simulink model "Param_Est_P1"  (R2019b)
settings: Solver=VariableStepAuto  StartTime=0.0  StopTime=50  RelTol=1e-3
undefined symbols (not defined in the file): sigbuilder_block
libraries: simulink x1
settings Model: Creator=Kevin  LastModifiedBy=Kevin

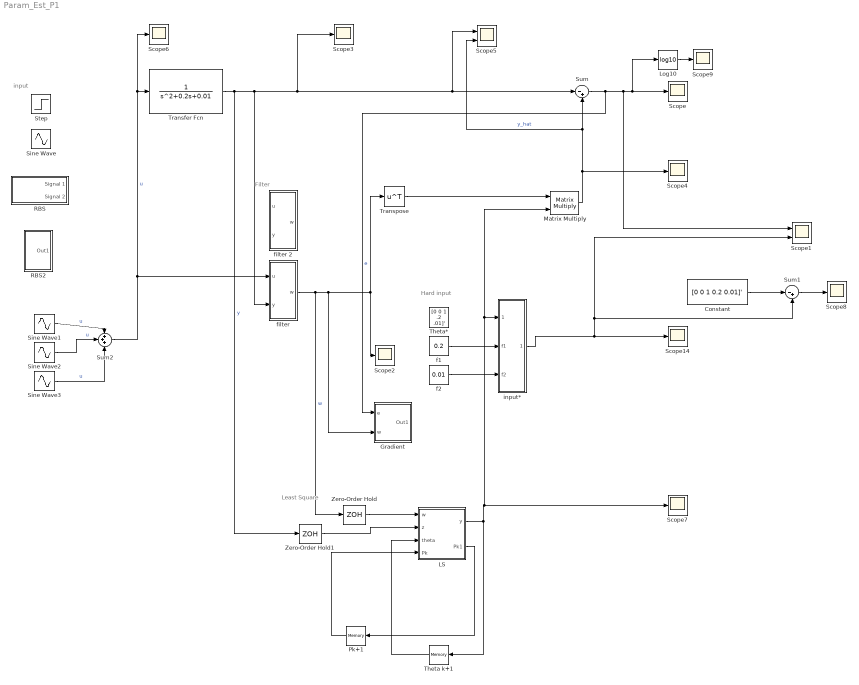
== system Param_Est_P1 ==
  note: Filter
  note: Least Square
  note: Hard input
  note: input
  Constant : Constant  Value=[0 0 1 0.2 0.01]'
  Gradient : Subsystem
  LS : MATLAB Function  TreatAsAtomicUnit=on
  Log10 : Math  Operator=log10  SignedPower=off  SaturateOnIntegerOverflow=on
  Matrix Multiply : Product  Multiplication=Matrix(*)
  Pk+1 : Memory  InitialCondition=(10^5)*eye(5)
  "RBS " : Subsystem  Tag=STV Subsys  LoadFcn=sigbuilder_block('load');  StartFcn=sigbuilder_block('start');  StopFcn=sigbuilder_block('stop');  ClipboardFcn=sigbuilder_block('clipboard');  mask(Sigbuilder block){tuvar=[0:10]}
      mask help: Simulink:masks:SigbuilderBlock_MD
      mask init:
      | if ~strcmp(get_param(bdroot(gcbh),'SimulationStatus'),'stopped') tuvar = sigbuilder_block('maskInit'); end
      settings: CopyFcn=sigbuilder_block('copy');  DeleteFcn=sigbuilder_block('delete');  ModelCloseFcn=sigbuilder_block('modelClose');  PreSaveFcn=sigbuilder_block('preSave');  PauseFcn=sigbuilder_block('pause');  ContinueFcn=sigbuilder_block('continue');  NameChangeFcn=sigbuilder_block('namechange');  OpenFcn=sigbuilder_block('open',[215 62.5 550.5 362.5 ]);  CloseFcn=sigbuilder_block('close');
      mask Display: plot(0, 0, 100, 100,[2, 2, 32, 32, 2], [68, 8, 8, 68, 68],[32, 2], [38, 38], [32, 19, 2],[53, 60, 44], [32, 17, 17, 2],[16, 16, 31, 31]);txt = getActiveGroup(gcbh);text(2, 100, txt,'verticalAlignment', 'top');
  RBS2 : Subsystem
  Scope{,2..4,6..9,14} (9 alike) : Scope
  Scope1 : Scope  NumInputPorts=2
  Scope5 : Scope  NumInputPorts=2
  Sine Wave : Sin  Frequency=0.1  SampleTime=0
  Sine Wave1 : Sin  Frequency=0.1  Phase=0.1  SampleTime=0
  Sine Wave2 : Sin  SampleTime=0
  Sine Wave3 : Sin  Frequency=2  SampleTime=0
  Step : Step  SampleTime=0
  Sum : Sum  Inputs=|-+
  Sum1 : Sum  Inputs=|-+
  Sum2 : Sum  Inputs=+++
  Theta k+1 : Memory  InitialCondition=[0 0 0 0 0]'
  Theta* : Constant  Value=[0 0 1 .2 .01]'
  Transfer Fcn : TransferFcn  Denominator=[1 ,0.2 ,0.01]
  Transpose : Math  Operator=transpose  SignedPower=off  SaturateOnIntegerOverflow=on
  Zero-Order Hold : ZeroOrderHold  SampleTime=-1
  Zero-Order Hold1 : ZeroOrderHold  SampleTime=-1
  f1 : Constant  Value=0.2
  f2 : Constant  Value=0.01
  "filter " : Subsystem
  filter 2 : Subsystem
  input* : Subsystem
  wires:
  "filter "/1(w) -> Zero-Order Hold/1, Gradient/2(w), Scope2/1, Transpose/1  "w"
  Matrix Multiply/1 -> Sum/2, Scope5/2, Scope4/1  "y_hat"
  Sum/1 -> Gradient/1(e), Scope1/1, Log10/1, Scope/1  "e"
  Transpose/1 -> Matrix Multiply/1
  f1/1 -> input*/2(f1)
  f2/1 -> input*/3(f2)
  Zero-Order Hold/1 -> LS/1(w)
  LS/1(y) -> Theta k+1/1, Matrix Multiply/2, input*/1(theta), Scope7/1
  Theta k+1/1 -> LS/3(theta)
  Pk+1/1 -> LS/4(Pk)
  LS/2(Pk1) -> Pk+1/1
  Transfer Fcn/1 -> Zero-Order Hold1/1, "filter "/2("y "), Scope5/1, Sum/1, Scope3/1  "y"
  Zero-Order Hold1/1 -> LS/2(z)
  Sum2/1 -> Transfer Fcn/1, Scope6/1, "filter "/1("u ")  "u"
  input*/1(Out1) -> Sum1/2, Scope1/2, Scope14/1
  Constant/1 -> Sum1/1
  Sum1/1 -> Scope8/1
  Sine Wave1/1 -> Sum2/1  "u"
  Sine Wave2/1 -> Sum2/2  "u"
  Sine Wave3/1 -> Sum2/3  "u"
  Log10/1 -> Scope9/1

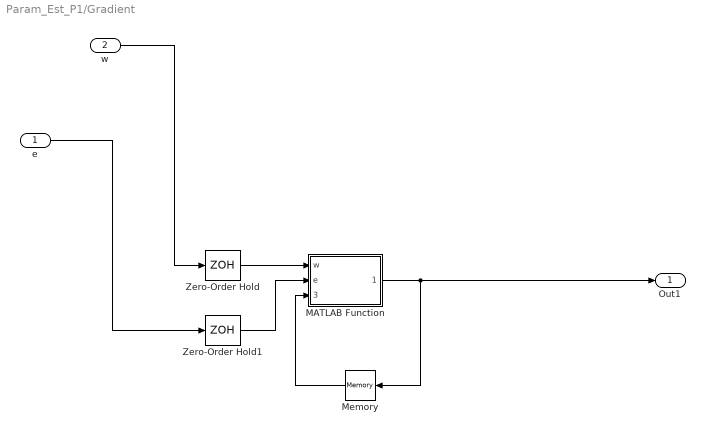
== system Param_Est_P1/Gradient ==
  e : Inport
  w : Inport  Port=2
  MATLAB Function : MATLAB Function  TreatAsAtomicUnit=on
  Memory : Memory  InitialCondition=[0 0 0.9 0.000001 0.0000001]'
  Zero-Order Hold : ZeroOrderHold  SampleTime=0.01
  Zero-Order Hold1 : ZeroOrderHold  SampleTime=0.01
  Out1 : Outport
  wires:
  MATLAB Function/1(theta_k1) -> Memory/1, Out1/1
  Zero-Order Hold/1 -> MATLAB Function/1(w)
  w/1 -> Zero-Order Hold/1
  Zero-Order Hold1/1 -> MATLAB Function/2(e)
  e/1 -> Zero-Order Hold1/1
  Memory/1 -> MATLAB Function/3(theta_1)

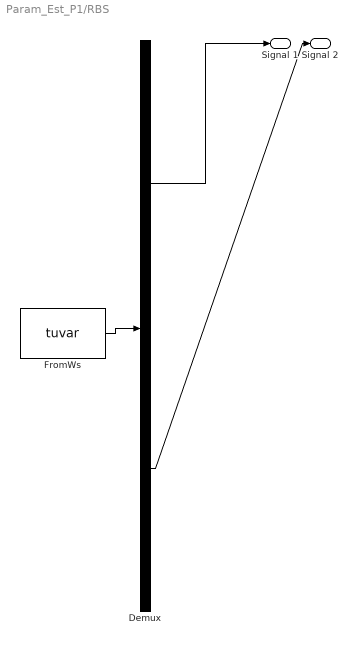
== system Param_Est_P1/RBS  ==
  Demux : Demux  Tag=STV Demux  Outputs=2
  FromWs : FromWorkspace  Tag=STV FromWs  VariableName=tuvar  SampleTime=0
      SigBuilderData=|
      | common.afterFinalStr = 'Extrapolate'
      | common.sampleTime = 0
      | dataSet.timeRange = [0 10]
      | dataSet.name = 'Group 1'
      | sbobj.Groups.Name = 'Group 1'
      | sbobj.Groups.Signals(1).Name = 'Signal 1'
      | sbobj.Groups.Signals(1).XData = [0 4 4 6 6 10]
      | sbobj.Groups.Signals(1).YData = [0 0 1 1 0 0]
      | sbobj.Groups.Signals(2).Name = 'Signal 2'
      | sbobj.Groups.Signals(2).XData = [0 0.2 0.2 0.3 0.3 0.5 0.5 0.7 0.7 1 1 1.1 1.1 1.3 1.3 1.4 1.4 1.5 1.5 1.7 1.7 2.1 2.1 2.2 2.2 2.7 2.7 2.8 2.8 2.9 2.9 3 3 3.1 3.1 3.5 3.5 3.7 3.7 3.8 3.8 3.9 3.9 4.2 4.2 4.4 4.4 4.7 4.7 5 5 5.1 5.1 5.3 5.3 5.6 5.6 5.7 5.7 5.8 5.8 5.9 5.9 6 6 6.1 6.1 6.2 6.2 6.7 6.7 7 7 7.1 7.1 7.2 7.2 7.3 7.3 7.4 7.4 7.5 7.5 7.8 7.8 7.9 7.9 8.1 8.1 8.5 8.5 8.6 8.6 8.8 8.8 8.9 8.9 9 9 9.2 9.2 9.5 9.5 9.6 9.6 9.7 9.7 10]
      | sbobj.Groups.Signals(2).YData = [1 1 0 0 1 1 0 0 1 1 0 0 1 1 0 0 1 1 0 0 1 1 0 0 1 1 0 0 1 1 0 0 1 1 0 0 1 1 0 0 1 1 0 0 1 1 0 0 1 1 0 0 1 1 0 0 1 1 0 0 1 1 0 0 1 1 0 0 1 1 0 0 1 1 0 0 1 1 0 0 1 1 0 0 1 1 0 0 1 1 0 0 1 1 0 0 1 1 0 0 1 1 0 0 1 1 0 0]
  Signal 1 : Outport  Tag=STV Outport
  Signal 2 : Outport  Tag=STV Outport  Port=2
  wires:
  Demux/1 -> Signal 1/1
  FromWs/1 -> Demux/1
  Demux/2 -> Signal 2/1

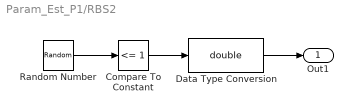
== system Param_Est_P1/RBS2 ==
  Compare To Constant : simulink/Logic and Bit Operations/Compare To Constant  relop=<=  const=1  OutDataTypeStr=boolean
  Data Type Conversion : DataTypeConversion  OutDataTypeStr=double
  Random Number : RandomNumber  Mean=1  SampleTime=10
  Out1 : Outport
  wires:
  Random Number/1 -> Compare To Constant/1
  Compare To Constant/1 -> Data Type Conversion/1
  Data Type Conversion/1 -> Out1/1

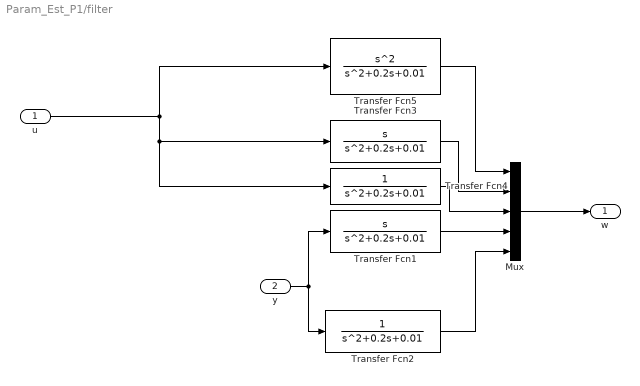
== system Param_Est_P1/filter  ==
  "u " : Inport
  "y " : Inport  Port=2
  Mux : Mux  Inputs=5
  Transfer Fcn1 : TransferFcn  Numerator=[1 0]  Denominator=[1 0.2 0.01]
  Transfer Fcn2 : TransferFcn  Denominator=[1 0.2 0.01]
  Transfer Fcn3 : TransferFcn  Numerator=[1 0]  Denominator=[1 0.2 0.01]
  Transfer Fcn4 : TransferFcn  Denominator=[1 0.2 0.01]
  Transfer Fcn5 : TransferFcn  Numerator=[1 0 0]  Denominator=[1 0.2 0.01]
  w : Outport
  wires:
  Transfer Fcn1/1 -> Mux/4
  "u "/1 -> Transfer Fcn4/1, Transfer Fcn3/1, Transfer Fcn5/1
  Mux/1 -> w/1
  "y "/1 -> Transfer Fcn1/1, Transfer Fcn2/1
  Transfer Fcn2/1 -> Mux/5
  Transfer Fcn5/1 -> Mux/1
  Transfer Fcn3/1 -> Mux/2
  Transfer Fcn4/1 -> Mux/3

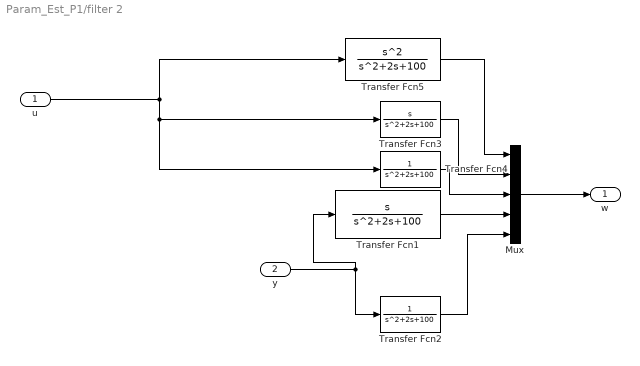
== system Param_Est_P1/filter 2 ==
  "u " : Inport
  "y " : Inport  Port=2
  Mux : Mux  Inputs=5
  Transfer Fcn1 : TransferFcn  Numerator=[1 0]  Denominator=[1 2 100]
  Transfer Fcn2 : TransferFcn  Denominator=[1 2 100]
  Transfer Fcn3 : TransferFcn  Numerator=[1 0]  Denominator=[1 2 100]
  Transfer Fcn4 : TransferFcn  Denominator=[1 2 100]
  Transfer Fcn5 : TransferFcn  Numerator=[1 0 0]  Denominator=[1 2 100]
  w : Outport
  wires:
  Transfer Fcn1/1 -> Mux/4
  "u "/1 -> Transfer Fcn4/1, Transfer Fcn3/1, Transfer Fcn5/1
  Mux/1 -> w/1
  "y "/1 -> Transfer Fcn2/1, Transfer Fcn1/1
  Transfer Fcn2/1 -> Mux/5
  Transfer Fcn5/1 -> Mux/1
  Transfer Fcn3/1 -> Mux/2
  Transfer Fcn4/1 -> Mux/3

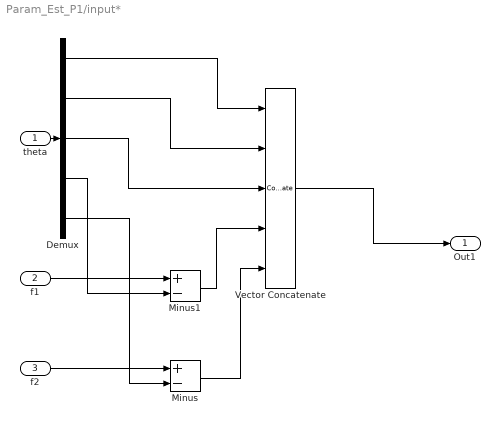
== system Param_Est_P1/input* ==
  theta : Inport
  f1 : Inport  Port=2
  f2 : Inport  Port=3
  Demux : Demux  Outputs=5
  Minus : Sum  Inputs=+-
  Minus1 : Sum  Inputs=+-
  Vector Concatenate : Concatenate  NumInputs=5
  Out1 : Outport
  wires:
  Vector Concatenate/1 -> Out1/1
  Minus1/1 -> Vector Concatenate/4
  Minus/1 -> Vector Concatenate/5
  Demux/1 -> Vector Concatenate/1
  Demux/4 -> Minus1/2
  Demux/3 -> Vector Concatenate/3
  Demux/5 -> Minus/2
  f2/1 -> Minus/1
  Demux/2 -> Vector Concatenate/2
  f1/1 -> Minus1/1
  theta/1 -> Demux/1

== matlab function Param_Est_P1/Gradient/MATLAB Function ==
  data: w input; theta_k1 output; e input; theta_1 input
function theta_k1 = fcn(w, e, theta_1)
gamma = 0.000001;
dt = 0.01;
%I = eye(5);
%gamma = alpha*I;
theta_dot = -gamma*w*e;
theta_k1 = theta_1 + theta_dot*dt;

== matlab function Param_Est_P1/LS ==
  data: w input; z input; theta input; Pk input; y output; Pk1 output
function [ y,Pk1] = fcn(w, z, theta, Pk)
alpha = 1; %standard
gamma = 1/alpha;
%e = 10^-4;
%Q = e*eye(5);
%Pk = eye(5);

%initial values
%ro = 10^5;
%P1 = ro*eye(5);
%theta1 = [0 0 1 0.2 0.01]';
%Calculations

theta_k1 = theta - (gamma*Pk*w*(w'*theta-z))/ (1+gamma*w'*Pk*w);
y = theta_k1;
Pk1 = (1/alpha)*Pk - ((gamma^2*Pk*w*w'*Pk)/(1+gamma*w'*Pk*w));
